simulink subsystem "Autopilot_Commands"  (R2023b)
settings: Solver=VariableStepAuto  StartTime=0.0  StopTime=10.0  RelTol=1e-3
undefined symbols (not defined in the file): Kd, KD_Lateral, Ki, KI_BCL, Kp, KP_BCL, KP_Lateral, KP_TECL, servoLimits
libraries: slpidlib x5, checkpacklib x3, simulink_extras x3, sharedtransform x2
settings Model: Creator=cyber  LastModifiedBy=cyber

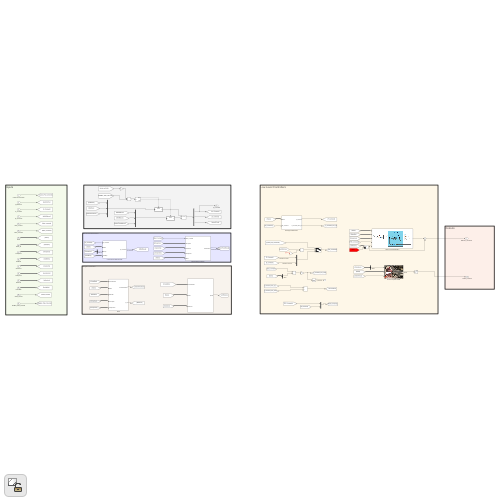
[thumbnail: Simulink's stored preview of the top-level diagram]
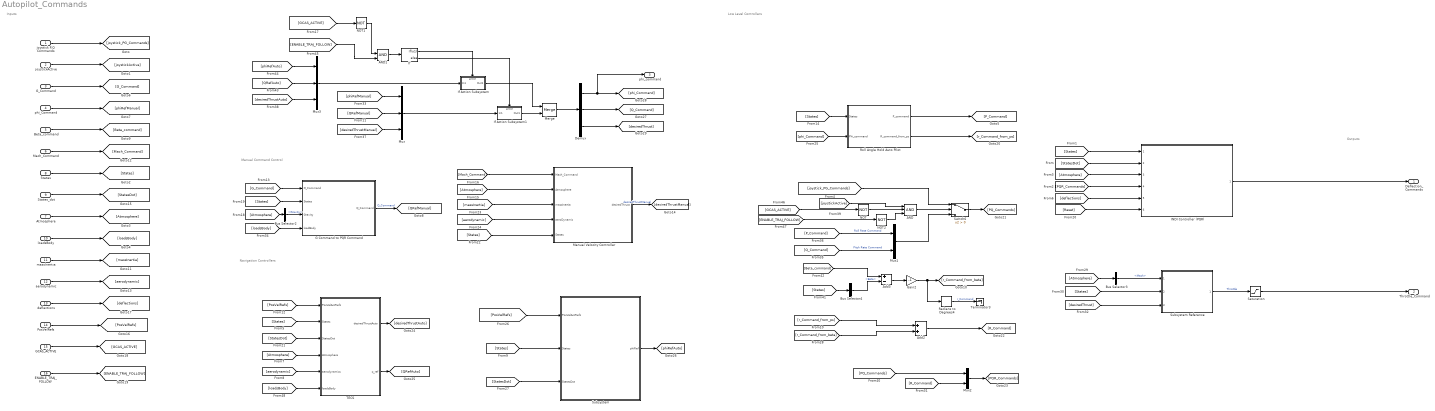
== system Autopilot_Commands ==
  note: Inputs
  note: Manual Command Control
  note: Low Level Controllers
  note: Navigation Controllers
  note: Outputs
  joystick P,Q Commands : Inport
  joystickActive : Inport  Port=2
  G_Command : Inport  Port=3
  phi_Command : Inport  Port=4
  Beta_command : Inport  Port=5
  Mach_Command : Inport  Port=6
  Atmosphere : Inport  Port=7
  States : Inport  Port=8
  States_dot : Inport  Port=9
  loadsBody : Inport  Port=10
  massInertıa : Inport  Port=11
  aerodynamic : Inport  Port=12
  deflections : Inport  Port=13
  PosVelRefs : Inport  Port=14
  GCAS_ACTIVE : Inport  Port=15
  ENABLE_TRAJ_FOLLOW : Inport  Port=16
  AND : Logic  Inputs=3  IconShape=distinctive  AllPortsSameDT=off  OutDataTypeStr=boolean
  AND1 : Logic  IconShape=distinctive  AllPortsSameDT=off  OutDataTypeStr=boolean
  Add2 : Sum
  Add3 : Sum  Inputs=+-
  Bus Selector2 : BusSelector  OutputSignals=Gravity
  Bus Selector3 : BusSelector  OutputSignals=Mach
  Bus Selector4 : BusSelector  OutputSignals=Beta
  Demux : Demux  Outputs=3
  G Command to PQR Command : Subsystem
  Gain2 : Gain  Gain=-1
  INDI Controller (PQR) : Subsystem  ReferencedSubsystem=INDI_Controller_PQR
  If : If  IfExpression=u1
  If Action Subsystem : Subsystem  TreatAsAtomicUnit=on
  If Action Subsystem1 : Subsystem  TreatAsAtomicUnit=on
  Manual Velocity Controller : Subsystem
  Merge : Merge
  Mux : Mux  Inputs=3
  Mux1 : Mux  Inputs=2
  Mux2 : Mux  Inputs=2
  Mux3 : Mux  Inputs=3
  NOT : Logic  Operator=NOT  IconShape=distinctive  AllPortsSameDT=off  OutDataTypeStr=boolean
  NOT1 : Logic  Operator=NOT  IconShape=distinctive  AllPortsSameDT=off  OutDataTypeStr=boolean
  NOT2 : Logic  Operator=NOT  IconShape=distinctive  AllPortsSameDT=off  OutDataTypeStr=boolean
  Radians to Degrees4 : simulink_extras/Transformations/Radians to Degrees
  "Roll Angle Hold Auto Pilot " : Subsystem
  Saturation : Saturate  UpperLimit=100  LowerLimit=-100
  Subsystem : Subsystem
  Subsystem Reference : Subsystem  ReferencedSubsystem=Reverse_Propulsion_Model
  Switch6 : Switch  Criteria=u2 > Threshold  SaturateOnIntegerOverflow=off  InputSameDT=off
  TECS : Subsystem
  Terminator3 : Terminator
  Deflection_Commands : Outport
  Throttle_Command : Outport  Port=2
  phi_command : Outport  Port=3
  wires:
  [PosVelRefs] -> TECS/1(PosVelAccRefs)
  Demux/3 -> [desiredThrust]
  [States] -> G Command to PQR Command/2(States)
  [aerodynamic] -> TECS/5(aerodynamics)
  Saturation/1 -> Throttle_Command/1
  Subsystem/1(phiRef) -> [phiRefAuto]
  If/1 -> If Action Subsystem/Action
  Add3/1 -> Gain2/1
  [phiRefAuto] -> Mux3/1
  [joystick_PG_Commands] -> Switch6/1
  Demux/1 -> [phi_Command], phi_command/1
  deflections/1 -> [deflections]
  [desiredThrustAuto] -> Mux3/3
  Merge/1 -> Demux/1
  If Action Subsystem1/1(Out1) -> Merge/2
  [States] -> "Roll Angle Hold Auto Pilot "/1(States)
  massInertıa/1 -> [massInertia]
  If/2 -> If Action Subsystem1/Action
  If Action Subsystem/1(Out1) -> Merge/1
  loadsBody/1 -> [loadsBody]
  [Mach_Command] -> Manual Velocity Controller/1(Mach_Command)
  [massInertia] -> Manual Velocity Controller/3(massInertia)
  AND1/1 -> If/1
  [States] -> Manual Velocity Controller/5(States)
  Demux/2 -> [Q_Command]
  Mux/1 -> If Action Subsystem1/1(In1)
  [Atmosphere] -> Bus Selector2/1
  Subsystem Reference/1 -> Saturation/1  "Throttle"
  Bus Selector2/1 -> G Command to PQR Command/3(Gravity)  "<Gravity>"
  [Q_Command] -> Mux1/2  "Pitch Rate Command"
  Bus Selector3/1 -> Subsystem Reference/1  "<Mach>"
  [States] -> Subsystem Reference/2
  [phiRefManual] -> Mux/1
  [R_Command] -> Mux2/2
  TECS/2(q_ref) -> [QRefAuto]
  G_Command/1 -> [G_Command]
  [Atmosphere] -> Bus Selector3/1
  [Atmosphere] -> Manual Velocity Controller/2(Atmosphere)
  aerodynamic/1 -> [aerodynamic]
  [PosVelRefs] -> Subsystem/1(PosVelAccRefs)
  G Command to PQR Command/1(Q_Command) -> [QRefManual]  "Q_Command"
  [States] -> Subsystem/2(States)
  [StatesDot] -> TECS/3(StatesDot)
  [Atmosphere] -> TECS/4(Atmosphere)
  Mach_Command/1 -> [Mach_Command]
  [QRefAuto] -> Mux3/2
  [StatesDot] -> Subsystem/3(StatesDot)
  Beta_command/1 -> [Beta_command]
  States_dot/1 -> [StatesDot]
  Switch6/1 -> [PQ_Commands]
  [desiredThrustManual] -> Mux/3
  Mux1/1 -> Switch6/3
  TECS/1(desiredThrustAuto) -> [desiredThrustAuto]
  [G_Command] -> G Command to PQR Command/1(G_Command)
  Atmosphere/1 -> [Atmosphere]
  Gain2/1 -> [r_Command_from_beta], Radians to Degrees4/1
  AND/1 -> Switch6/2
  [P_Command] -> Mux1/1  "Roll Rate Command"
  [loadsBody] -> G Command to PQR Command/4(loadBody)
  States/1 -> [States]
  [desiredThrust] -> Subsystem Reference/3
  joystick P,Q Commands/1 -> [joystick_PG_Commands]
  joystickActive/1 -> [joystickActive]
  phi_Command/1 -> [phiRefManual]
  PosVelRefs/1 -> [PosVelRefs]
  [States] -> TECS/2(States)
  Manual Velocity Controller/1(desiredThrust) -> [desiredThrustManual]  "desiredThrustManual"
  Bus Selector4/1 -> Add3/2  "<Beta>"
  [phi_Command] -> "Roll Angle Hold Auto Pilot "/2(Phi_command)
  "Roll Angle Hold Auto Pilot "/2(R_command_from_ps) -> [r_Command_from_ps]
  [r_Command_from_beta] -> Add2/2
  [QRefManual] -> Mux/2
  [PQ_Commands] -> Mux2/1
  Mux3/1 -> If Action Subsystem/1(In1)
  Add2/1 -> [R_Command]
  "Roll Angle Hold Auto Pilot "/1(P_command) -> [P_Command]
  Radians to Degrees4/1 -> Terminator3/1  "r_Command"
  [States] -> Bus Selector4/1
  [aerodynamic] -> Manual Velocity Controller/4(aeroDynamic)
  [r_Command_from_ps] -> Add2/1
  [Beta_command] -> Add3/1
  Mux2/1 -> [PQR_Commands]
  [GCAS_ACTIVE] -> NOT/1
  NOT/1 -> AND/2
  [joystickActive] -> AND/1
  GCAS_ACTIVE/1 -> [GCAS_ACTIVE]
  [GCAS_ACTIVE] -> NOT1/1
  ENABLE_TRAJ_FOLLOW/1 -> [ENABLE_TRAJ_FOLLOW]
  NOT1/1 -> AND1/1
  [ENABLE_TRAJ_FOLLOW] -> AND1/2
  [ENABLE_TRAJ_FOLLOW] -> NOT2/1
  NOT2/1 -> AND/3
  [loadsBody] -> TECS/6(loadsBody)
  [States] -> INDI Controller (PQR)/1
  [StatesDot] -> INDI Controller (PQR)/2
  [Atmosphere] -> INDI Controller (PQR)/3
  [PQR_Commands] -> INDI Controller (PQR)/4
  [deflections] -> INDI Controller (PQR)/5
  [Reset] -> INDI Controller (PQR)/6
  INDI Controller (PQR)/1 -> Deflection_Commands/1

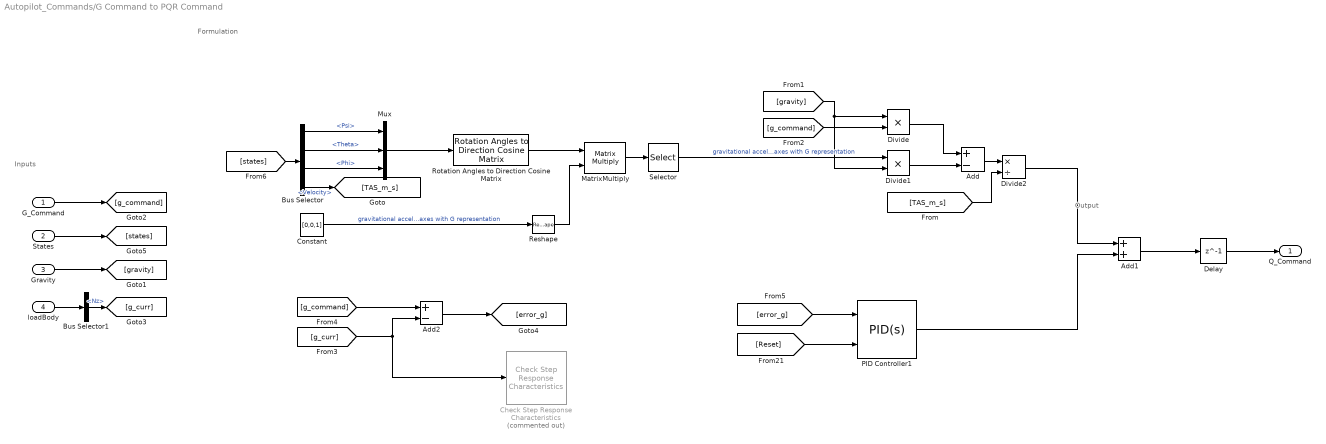
== system Autopilot_Commands/G Command to PQR Command ==
  note: Formulation
  note: Output
  note: Inputs
  G_Command : Inport
  States : Inport  Port=2
  Gravity : Inport  Port=3
  loadBody : Inport  Port=4
  Add : Sum  Inputs=+-
  Add1 : Sum
  Add2 : Sum  Inputs=+-
  Bus Selector : BusSelector  OutputSignals=Psi,Theta,Phi,Velocity
  Bus Selector1 : BusSelector  OutputSignals=Nz
  Check Step Response Characteristics : checkpacklib/Check Step Response  Characteristics  Commented=on  InstantiateOnLoad=on  enabled=off  stopWhenAssertionFail=off  export=off  ViewDlgPos=[]  OpenViewOnLoad=off  LaunchViewOnOpen=off  TimeUnits=seconds  EnableStepResponseBound=on  InitialValue=1  FinalValue=5  StepTime=0  RiseTime=0.5  PercentRise=90  SettlingTime=1.2  PercentSettling=1  PercentOvershoot=5  PercentUndershoot=1
      settings: LibrarySourceBlock=|
      | sdolib/Model Verification/Check Step Response
      | Characteristics
  Constant : Constant  Value=[0,0,1]
  Delay : Delay  DelayLength=1
  Divide : Product  Inputs=**
  Divide1 : Product  Inputs=**
  Divide2 : Product  Inputs=*/
  MatrixMultiply : Product  Multiplication=Matrix(*)
  Mux : Mux  Inputs=3
  PID Controller1 : slpidlib/PID Controller  Controller=PID  Form=Parallel  TimeDomain=Continuous-time  UseExternalTs=off  SampleTime=-1  IntegratorMethod=Forward Euler  FilterMethod=Forward Euler  ControllerParametersSource=internal  P=Kp  I=Ki  UseKiTs=off  D=Kd  N=100  UseFilter=on  TunerSelectOption=Transfer Function Based (PID Tuner App)  InitialConditionSource=internal  InitialConditionForIntegrator=0  InitialConditionForFilter=0  DifferentiatorICPrevScaledInput=0  ExternalReset=either  TrackingMode=off  Kt=1  LimitOutput=off  SatLimitsSource=external  UpperSaturationLimit=inf  LowerSaturationLimit=-inf  LinearizeAsGain=on  AntiWindupMode=clamping  Kb=1  LimitIntegrator=off  UpperIntegratorSaturationLimit=inf  LowerIntegratorSaturationLimit=-inf  POutMin=[]  POutMax=[]  IOutMin=[]  IOutMax=[]  DOutMin=[]  DOutMax=[]  NOutMin=[]  NOutMax=[]  SumOutMin=[]  SumOutMax=[]  SaturationOutMin=[]  SaturationOutMax=[]  PParamMin=[]  PParamMax=[]  IParamMin=[]  IParamMax=[]  DParamMin=[]  DParamMax=[]  NParamMin=[]  NParamMax=[]  KbParamMin=[]  KbParamMax=[]  KtParamMin=[]  KtParamMax=[]  KbOutMin=[]  KbOutMax=[]  KtOutMin=[]  KtOutMax=[]  IntegratorOutMin=[]  IntegratorOutMax=[]  FilterOutMin=[]  FilterOutMax=[]  SumI1OutMin=[]  SumI1OutMax=[]  SumI2OutMin=[]  SumI2OutMax=[]  SumI3OutMin=[]  SumI3OutMax=[]  SumI4OutMin=[]  SumI4OutMax=[]  SumDOutMin=[]  SumDOutMax=[]  DifferentiatorOutMin=[]  DifferentiatorOutMax=[]  FilterDiffOutCoefMin=[]  FilterDiffOutCoefMax=[]  ReciprocalOutMin=[]  ReciprocalOutMax=[]  SumDenOutMin=[]  SumDenOutMax=[]  SumNumOutMin=[]  SumNumOutMax=[]  DivideOutMin=[]  DivideOutMax=[]  UdiffTsProdOutMin=[]  UdiffTsProdOutMax=[]  NTsProdOutMin=[]  NTsProdOutMax=[]  UintegralTsProdOutMin=[]  UintegralTsProdOutMax=[]  UngainTsProdOutMin=[]  UngainTsProdOutMax=[]  ClampingZeroOutDataTypeStr=Inherit: Inherit via back propagation  ClampingZeroOutMin=[]  ClampingZeroOutMax=[]  FilterDenConstantOutDataTypeStr=Inherit: Inherit via back propagation  FilterDenConstantOutMin=[]  FilterDenConstantOutMax=[]  PCopyOutDataTypeStr=Inherit: Inherit via back propagation  PCopyOutMin=[]  PCopyOutMax=[]  NCopyOutDataTypeStr=Inherit: Inherit via back propagation  NCopyOutMin=[]  NCopyOutMax=[]  IntegratorContinuousStateAttributes=''  IntegratorStateMustResolveToSignalObject=off  IntegratorRTWStateStorageClass=Auto  FilterContinuousStateAttributes=''  FilterStateMustResolveToSignalObject=off  FilterRTWStateStorageClass=Auto  ParallelPVariant=InternalParameters  IdealPVariant=Disabled  IVariant=InternalParameters  DVariant=InternalParameters  IntegratorVariant=Continuous  SatVariant=Disabled  AWVariant=Passthrough  PCopyVariant=Disabled  TRVariant=Disabled  FdbkBlocksVariant=Forward  IdealPFdbkVariant=Disabled  SatFdbkVariant=Disabled  DerivativeFilterVariant=ContFilter  NVariant=InternalParameters  NCopyVariant=Disabled  FilterICVariant=InternalICsFilter  IntegratorICVariant=InternalICs  ExternalResetVariant=ExternalReset  TRSumVariant=Passthrough  SumFdbkVariant=Disabled  SumVariant=Sum_PID  TsampFilterVariant=InternalTs  TsampNgainVariant=Passthrough  TsampIntegralVariant=Disabled_SignalSpec  ExternalSaturationOutDataTypeStr=Inherit: Same as second input
  Reshape : Reshape  OutputDimensionality=Column vector (2-D)
  Rotation Angles to Direction Cosine Matrix : sharedtransform/Rotation Angles to Direction Cosine Matrix  rotationOrder=ZYX  aMode=aMode
  Selector : Selector  InputPortWidth=3  IndexOptions=Index vector (dialog)  Indices=3  OutputSizes=1
  Q_Command : Outport
  wires:
  [states] -> Bus Selector/1
  Delay/1 -> Q_Command/1
  Add2/1 -> [error_g]
  [g_curr] -> Add2/2, Check Step Response Characteristics/1
  [g_command] -> Add2/1
  Bus Selector1/1 -> [g_curr]  "<Nz>"
  loadBody/1 -> Bus Selector1/1
  Add1/1 -> Delay/1
  PID Controller1/1 -> Add1/2
  [Reset] -> PID Controller1/2
  [error_g] -> PID Controller1/1
  G_Command/1 -> [g_command]
  Gravity/1 -> [gravity]
  Divide2/1 -> Add1/1
  Divide1/1 -> Add/2
  Divide/1 -> Add/1
  Selector/1 -> Divide1/1  "gravitational acceleration on Body Z axes with G representation"
  Add/1 -> Divide2/1
  [gravity] -> Divide1/2, Divide/1
  Reshape/1 -> MatrixMultiply/2
  [TAS_m_s] -> Divide2/2
  Bus Selector/4 -> [TAS_m_s]  "<Velocity>"
  [g_command] -> Divide/2
  MatrixMultiply/1 -> Selector/1
  Constant/1 -> Reshape/1  "gravitational acceleration on NED axes with G representation"
  Bus Selector/3 -> Mux/3  "<Phi>"
  Bus Selector/1 -> Mux/1  "<Psi>"
  Bus Selector/2 -> Mux/2  "<Theta>"
  Rotation Angles to Direction Cosine Matrix/1 -> MatrixMultiply/1
  Mux/1 -> Rotation Angles to Direction Cosine Matrix/1
  States/1 -> [states]

== system Autopilot_Commands/If Action Subsystem ==
  In1 : Inport
  Action Port : ActionPort
  Out1 : Outport
  wires:
  In1/1 -> Out1/1

== system Autopilot_Commands/If Action Subsystem1 ==
  In1 : Inport
  Action Port : ActionPort
  Out1 : Outport
  wires:
  In1/1 -> Out1/1

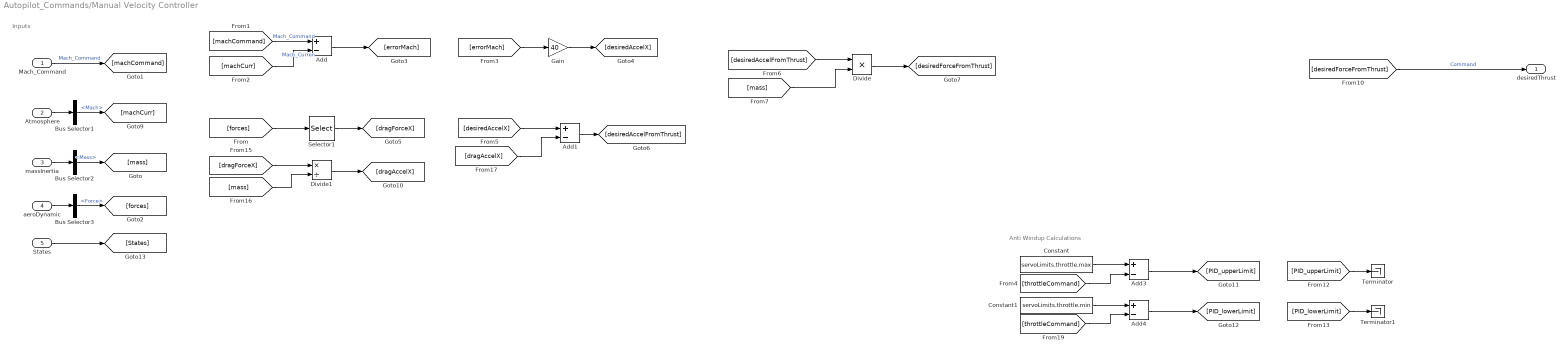
== system Autopilot_Commands/Manual Velocity Controller ==
  note: Inputs
  note: Anti Windup Calculations
  Mach_Command : Inport
  Atmosphere : Inport  Port=2
  massInertia : Inport  Port=3
  aeroDynamic : Inport  Port=4
  States : Inport  Port=5
  Add{,1,3..4} (4 alike) : Sum  Inputs=+-
  Bus Selector1 : BusSelector  OutputSignals=Mach
  Bus Selector2 : BusSelector  OutputSignals=Mass
  Bus Selector3 : BusSelector  OutputSignals=Force
  Constant : Constant  Value=servoLimits.throttle.max
  Constant1 : Constant  Value=servoLimits.throttle.min
  Divide : Product  Inputs=**
  Divide1 : Product  Inputs=*/
  Gain : Gain  Gain=40
  Selector1 : Selector  InputPortWidth=3  IndexOptions=Index vector (dialog)  Indices=1  OutputSizes=1
  Terminator : Terminator
  Terminator1 : Terminator
  desiredThrust : Outport
  wires:
  [PID_lowerLimit] -> Terminator1/1
  [PID_upperLimit] -> Terminator/1
  Atmosphere/1 -> Bus Selector1/1
  Bus Selector1/1 -> [machCurr]  "<Mach>"
  Mach_Command/1 -> [machCommand]  "Mach_Command"
  massInertia/1 -> Bus Selector2/1
  Bus Selector2/1 -> [mass]  "<Mass>"
  aeroDynamic/1 -> Bus Selector3/1
  Bus Selector3/1 -> [forces]  "<Force>"
  [forces] -> Selector1/1
  [machCurr] -> Add/2  "Mach_Curren"
  [machCommand] -> Add/1  "Mach_Command"
  Add/1 -> [errorMach]
  [errorMach] -> Gain/1
  Gain/1 -> [desiredAccelX]
  Selector1/1 -> [dragForceX]
  [desiredAccelX] -> Add1/1
  [dragAccelX] -> Add1/2
  Add1/1 -> [desiredAccelFromThrust]
  [desiredAccelFromThrust] -> Divide/1
  [mass] -> Divide/2
  Divide/1 -> [desiredForceFromThrust]
  States/1 -> [States]
  [dragForceX] -> Divide1/1
  [mass] -> Divide1/2
  Divide1/1 -> [dragAccelX]
  Constant1/1 -> Add4/1
  [throttleCommand] -> Add4/2
  [throttleCommand] -> Add3/2
  Constant/1 -> Add3/1
  Add4/1 -> [PID_lowerLimit]
  Add3/1 -> [PID_upperLimit]
  [desiredForceFromThrust] -> desiredThrust/1  "Command"

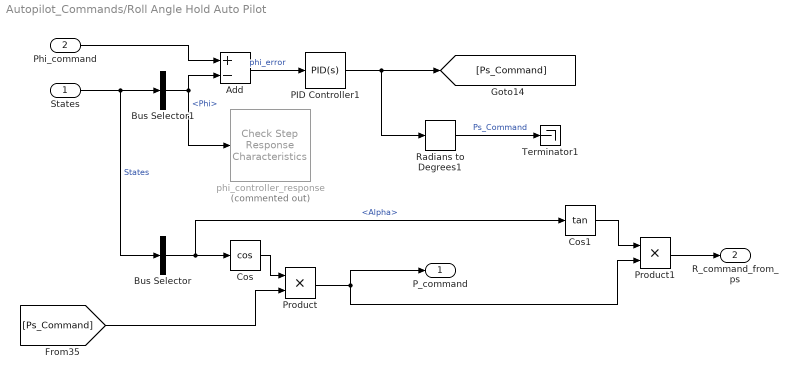
== system Autopilot_Commands/Roll Angle Hold Auto Pilot  ==
  States : Inport
  Phi_command : Inport  Port=2
  Add : Sum  Inputs=+-
  Bus Selector : BusSelector  OutputSignals=Alpha
  Bus Selector1 : BusSelector  OutputSignals=Phi
  Cos : Trigonometry  Operator=cos
  Cos1 : Trigonometry  Operator=tan
  PID Controller1 : slpidlib/PID Controller  Controller=PID  Form=Parallel  TimeDomain=Continuous-time  UseExternalTs=off  SampleTime=-1  IntegratorMethod=Forward Euler  FilterMethod=Forward Euler  ControllerParametersSource=internal  P=1.5  I=0  UseKiTs=off  D=5  N=0  UseFilter=on  TunerSelectOption=Transfer Function Based (PID Tuner App)  InitialConditionSource=internal  InitialConditionForIntegrator=0  InitialConditionForFilter=0  DifferentiatorICPrevScaledInput=0  ExternalReset=none  TrackingMode=off  Kt=1  LimitOutput=off  SatLimitsSource=internal  UpperSaturationLimit=inf  LowerSaturationLimit=-inf  LinearizeAsGain=on  AntiWindupMode=none  Kb=1  LimitIntegrator=off  UpperIntegratorSaturationLimit=inf  LowerIntegratorSaturationLimit=-inf  POutMin=[]  POutMax=[]  IOutMin=[]  IOutMax=[]  DOutMin=[]  DOutMax=[]  NOutMin=[]  NOutMax=[]  SumOutMin=[]  SumOutMax=[]  SaturationOutMin=[]  SaturationOutMax=[]  PParamMin=[]  PParamMax=[]  IParamMin=[]  IParamMax=[]  DParamMin=[]  DParamMax=[]  NParamMin=[]  NParamMax=[]  KbParamMin=[]  KbParamMax=[]  KtParamMin=[]  KtParamMax=[]  KbOutMin=[]  KbOutMax=[]  KtOutMin=[]  KtOutMax=[]  IntegratorOutMin=[]  IntegratorOutMax=[]  FilterOutMin=[]  FilterOutMax=[]  SumI1OutMin=[]  SumI1OutMax=[]  SumI2OutMin=[]  SumI2OutMax=[]  SumI3OutMin=[]  SumI3OutMax=[]  SumI4OutMin=[]  SumI4OutMax=[]  SumDOutMin=[]  SumDOutMax=[]  DifferentiatorOutMin=[]  DifferentiatorOutMax=[]  FilterDiffOutCoefMin=[]  FilterDiffOutCoefMax=[]  ReciprocalOutMin=[]  ReciprocalOutMax=[]  SumDenOutMin=[]  SumDenOutMax=[]  SumNumOutMin=[]  SumNumOutMax=[]  DivideOutMin=[]  DivideOutMax=[]  UdiffTsProdOutMin=[]  UdiffTsProdOutMax=[]  NTsProdOutMin=[]  NTsProdOutMax=[]  UintegralTsProdOutMin=[]  UintegralTsProdOutMax=[]  UngainTsProdOutMin=[]  UngainTsProdOutMax=[]  ClampingZeroOutDataTypeStr=Inherit: Inherit via back propagation  ClampingZeroOutMin=[]  ClampingZeroOutMax=[]  FilterDenConstantOutDataTypeStr=Inherit: Inherit via back propagation  FilterDenConstantOutMin=[]  FilterDenConstantOutMax=[]  PCopyOutDataTypeStr=Inherit: Inherit via back propagation  PCopyOutMin=[]  PCopyOutMax=[]  NCopyOutDataTypeStr=Inherit: Inherit via back propagation  NCopyOutMin=[]  NCopyOutMax=[]  IntegratorContinuousStateAttributes=''  IntegratorStateMustResolveToSignalObject=off  IntegratorRTWStateStorageClass=Auto  FilterContinuousStateAttributes=''  FilterStateMustResolveToSignalObject=off  FilterRTWStateStorageClass=Auto  ParallelPVariant=InternalParameters  IdealPVariant=Disabled  IVariant=InternalParameters  DVariant=InternalParameters  IntegratorVariant=Continuous  SatVariant=Disabled  AWVariant=Passthrough  PCopyVariant=Disabled  TRVariant=Disabled  FdbkBlocksVariant=Forward  IdealPFdbkVariant=Disabled  SatFdbkVariant=Disabled  DerivativeFilterVariant=ContFilter  NVariant=InternalParameters  NCopyVariant=Disabled  FilterICVariant=InternalICsFilter  IntegratorICVariant=InternalICs  ExternalResetVariant=Disabled  TRSumVariant=Passthrough  SumFdbkVariant=Disabled  SumVariant=Sum_PID  TsampFilterVariant=InternalTs  TsampNgainVariant=Passthrough  TsampIntegralVariant=Disabled_SignalSpec  ExternalSaturationOutDataTypeStr=Inherit: Same as second input
  Product : Product
  Product1 : Product
  Radians to Degrees1 : simulink_extras/Transformations/Radians to Degrees
  Terminator1 : Terminator
  phi_controller_response : checkpacklib/Check Step Response  Characteristics  Commented=on  InstantiateOnLoad=on  enabled=off  stopWhenAssertionFail=off  export=off  ViewDlgPos=[]  OpenViewOnLoad=off  LaunchViewOnOpen=off  TimeUnits=seconds  EnableStepResponseBound=on  InitialValue=0  FinalValue=pi/2  StepTime=0  RiseTime=2  PercentRise=90  SettlingTime=3  PercentSettling=2  PercentOvershoot=3  PercentUndershoot=1
      settings: LibrarySourceBlock=|
      | sdolib/Model Verification/Check Step Response
      | Characteristics
  P_command : Outport
  R_command_from_ps : Outport  Port=2
  wires:
  Product1/1 -> R_command_from_ps/1
  Add/1 -> PID Controller1/1  "phi_error"
  Bus Selector1/1 -> Add/2, phi_controller_response/1  "<Phi>"
  Cos/1 -> Product/1
  Bus Selector/1 -> Cos/1, Cos1/1  "<Alpha>"
  Phi_command/1 -> Add/1
  Radians to Degrees1/1 -> Terminator1/1  "Ps_Command"
  Cos1/1 -> Product1/1
  Product/1 -> Product1/2, P_command/1
  PID Controller1/1 -> Radians to Degrees1/1, [Ps_Command]
  States/1 -> Bus Selector1/1, Bus Selector/1  "States"
  [Ps_Command] -> Product/2

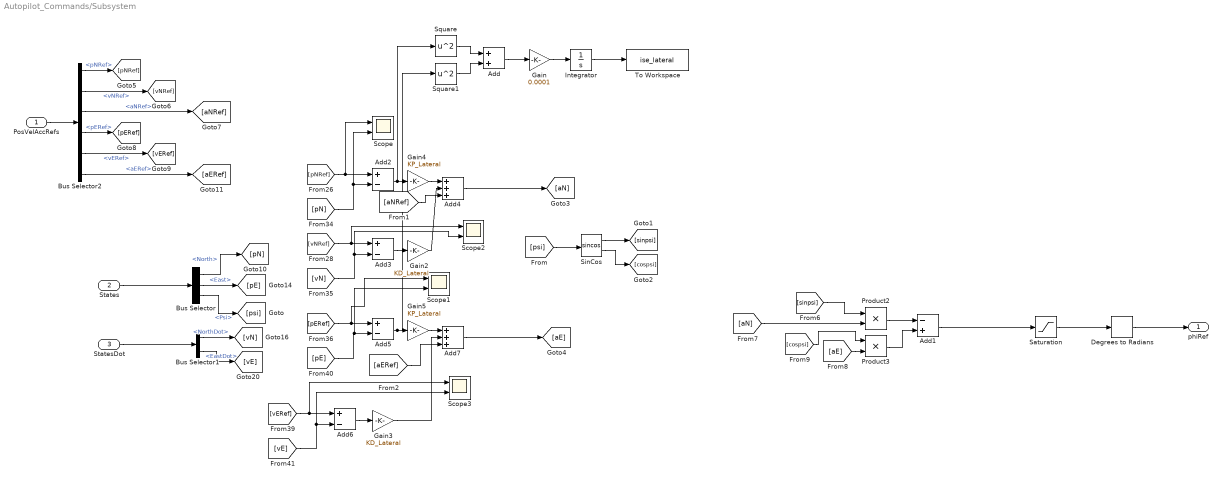
== system Autopilot_Commands/Subsystem ==
  PosVelAccRefs : Inport
  States : Inport  Port=2
  StatesDot : Inport  Port=3
  Add : Sum
  Add1 : Sum  Inputs=-+
  Add{2..3,5..6} (4 alike) : Sum  Inputs=+-
  Add4 : Sum  Inputs=+++
  Add7 : Sum  Inputs=+++
  Bus Selector : BusSelector  OutputSignals=North,East,Psi
  Bus Selector1 : BusSelector  OutputSignals=NorthDot,EastDot
  Bus Selector2 : BusSelector  OutputSignals=pNRef,vNRef,aNRef,pERef,vERef,aERef
  Degrees to Radians : simulink_extras/Transformations/Degrees to Radians
  Gain : Gain  Gain=0.0001
  Gain2 : Gain  Gain=KD_Lateral
  Gain3 : Gain  Gain=KD_Lateral
  Gain4 : Gain  Gain=KP_Lateral
  Gain5 : Gain  Gain=KP_Lateral
  Integrator : Integrator
  Product2 : Product
  Product3 : Product
  Saturation : Saturate  UpperLimit=60  LowerLimit=-60
  Scope{,1..3} (4 alike) : Scope  NumInputPorts=2
  SinCos : Trigonometry  Operator=sincos
  Square : Math  Operator=square
  Square1 : Math  Operator=square
  To Workspace : ToWorkspace  VariableName=ise_lateral  SaveFormat=Timeseries  SampleTime=-1
  phiRef : Outport
  wires:
  [aERef] -> Add7/3
  [aNRef] -> Add4/3
  Bus Selector2/6 -> [aERef]  "<aERef>"
  Bus Selector2/5 -> [vERef]  "<vERef>"
  Bus Selector2/4 -> [pERef]  "<pERef>"
  Bus Selector2/3 -> [aNRef]  "<aNRef>"
  Bus Selector2/2 -> [vNRef]  "<vNRef>"
  Bus Selector2/1 -> [pNRef]  "<pNRef>"
  PosVelAccRefs/1 -> Bus Selector2/1
  Add1/1 -> Saturation/1
  Gain/1 -> Integrator/1
  Integrator/1 -> To Workspace/1
  Square1/1 -> Add/2
  Square/1 -> Add/1
  Add/1 -> Gain/1
  Gain5/1 -> Add7/1
  Gain4/1 -> Add4/1
  Degrees to Radians/1 -> phiRef/1
  [pERef] -> Add5/1, Scope1/1
  [pE] -> Add5/2, Scope1/2
  Gain3/1 -> Add7/2
  Gain2/1 -> Add4/2
  Add4/1 -> [aN]
  Saturation/1 -> Degrees to Radians/1
  [aN] -> Product2/2
  [sinpsi] -> Product2/1
  [aE] -> Product3/2
  Product2/1 -> Add1/1
  [cospsi] -> Product3/1
  Product3/1 -> Add1/2
  SinCos/2 -> [cospsi]
  SinCos/1 -> [sinpsi]
  [psi] -> SinCos/1
  Bus Selector/3 -> [psi]  "<Psi>"
  StatesDot/1 -> Bus Selector1/1
  States/1 -> Bus Selector/1
  Bus Selector/1 -> [pN]  "<North>"
  Add5/1 -> Gain5/1, Square1/1
  [vERef] -> Add6/1, Scope3/1
  [vE] -> Add6/2, Scope3/2
  Bus Selector1/1 -> [vN]  "<NorthDot>"
  [pNRef] -> Add2/1, Scope/1
  [vNRef] -> Add3/1, Scope2/1
  [pN] -> Add2/2, Scope/2
  Bus Selector/2 -> [pE]  "<East>"
  [vN] -> Add3/2, Scope2/2
  Add6/1 -> Gain3/1
  Add3/1 -> Gain2/1
  Add7/1 -> [aE]
  Bus Selector1/2 -> [vE]  "<EastDot>"
  Add2/1 -> Gain4/1, Square/1

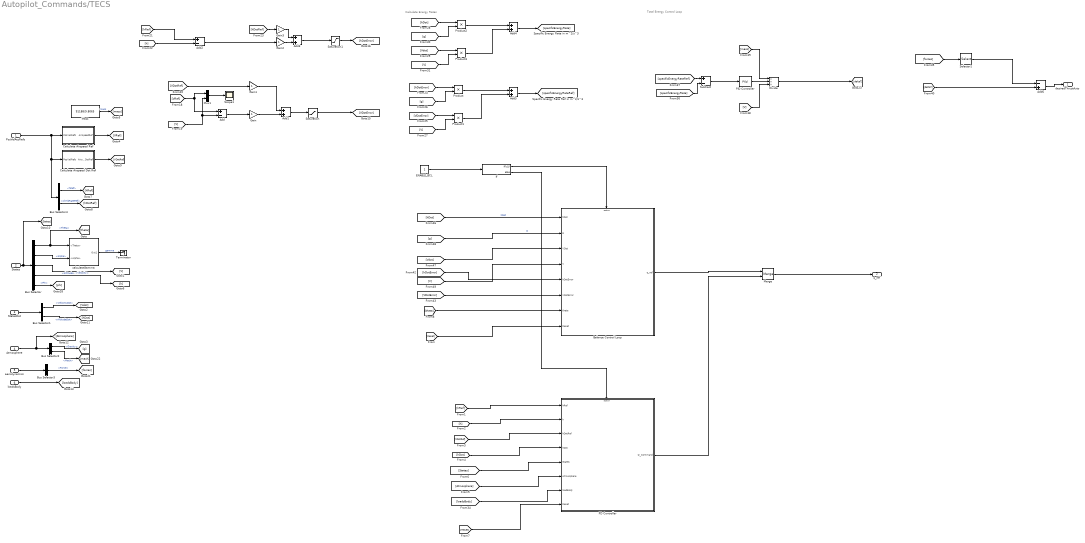
== system Autopilot_Commands/TECS ==
  note: Calculate Energy Rates
  note: Total Energy Control Loop
  PosVelAccRefs : Inport
  States : Inport  Port=2
  StatesDot : Inport  Port=3
  Atmosphere : Inport  Port=4
  aerodynamics : Inport  Port=5
  loadsBody : Inport  Port=6
  Add : Sum  Inputs=+-
  Add{1,3..5} (4 alike) : Sum
  Add2 : Sum  Inputs=+-
  Add6 : Sum  Inputs=-+
  Balance Control Loop : Subsystem
  Bus Selector : BusSelector  OutputSignals=Theta,Alpha,Velocity,Altitude,Phi
  Bus Selector1 : BusSelector  OutputSignals=VelocityDot,AltitudeDot
  Bus Selector2 : BusSelector  OutputSignals=Gravity,Mach
  Bus Selector3 : BusSelector  OutputSignals=Force
  Bus Selector4 : BusSelector  OutputSignals=hRef,climbRateRef
  Calculate Airspeed Dot Ref : Subsystem
  Calculate Airspeed Ref : Subsystem
  Divide : Product  Inputs=**/
  ENABLE_BCL : Constant
      settings: OpenFcn=|
      | val = get_param(gcb,'Value')
      | 
      | switch val
      | case '1'
      | set_param(gcb,'Value','0')
      | set_param(gcb,'BackGroundColor','red')
      | otherwise
      | set_param(gcb,'Value','1')
      | set_param(gcb,'BackGroundColor','green')
      | end
  Gain{,1..3} (4 alike) : Gain
  If : If  IfExpression=u1
  Mass : Constant  Value=91188/9.8065
  Merge : Merge
  Mux1 : Mux  Inputs=2
  PD Controller : Subsystem
  PID Controller : slpidlib/PID Controller  Controller=PI  Form=Parallel  TimeDomain=Continuous-time  UseExternalTs=off  SampleTime=-1  IntegratorMethod=Forward Euler  FilterMethod=Forward Euler  ControllerParametersSource=internal  P=KP_TECL  I=0  UseKiTs=off  D=0  N=100  UseFilter=on  TunerSelectOption=Transfer Function Based (PID Tuner App)  InitialConditionSource=internal  InitialConditionForIntegrator=0  InitialConditionForFilter=0  DifferentiatorICPrevScaledInput=0  ExternalReset=none  TrackingMode=off  Kt=1  LimitOutput=off  SatLimitsSource=internal  UpperSaturationLimit=inf  LowerSaturationLimit=-inf  LinearizeAsGain=on  AntiWindupMode=none  Kb=1  LimitIntegrator=off  UpperIntegratorSaturationLimit=inf  LowerIntegratorSaturationLimit=-inf  POutMin=[]  POutMax=[]  IOutMin=[]  IOutMax=[]  DOutMin=[]  DOutMax=[]  NOutMin=[]  NOutMax=[]  SumOutMin=[]  SumOutMax=[]  SaturationOutMin=[]  SaturationOutMax=[]  PParamMin=[]  PParamMax=[]  IParamMin=[]  IParamMax=[]  DParamMin=[]  DParamMax=[]  NParamMin=[]  NParamMax=[]  KbParamMin=[]  KbParamMax=[]  KtParamMin=[]  KtParamMax=[]  KbOutMin=[]  KbOutMax=[]  KtOutMin=[]  KtOutMax=[]  IntegratorOutMin=[]  IntegratorOutMax=[]  FilterOutMin=[]  FilterOutMax=[]  SumI1OutMin=[]  SumI1OutMax=[]  SumI2OutMin=[]  SumI2OutMax=[]  SumI3OutMin=[]  SumI3OutMax=[]  SumI4OutMin=[]  SumI4OutMax=[]  SumDOutMin=[]  SumDOutMax=[]  DifferentiatorOutMin=[]  DifferentiatorOutMax=[]  FilterDiffOutCoefMin=[]  FilterDiffOutCoefMax=[]  ReciprocalOutMin=[]  ReciprocalOutMax=[]  SumDenOutMin=[]  SumDenOutMax=[]  SumNumOutMin=[]  SumNumOutMax=[]  DivideOutMin=[]  DivideOutMax=[]  UdiffTsProdOutMin=[]  UdiffTsProdOutMax=[]  NTsProdOutMin=[]  NTsProdOutMax=[]  UintegralTsProdOutMin=[]  UintegralTsProdOutMax=[]  UngainTsProdOutMin=[]  UngainTsProdOutMax=[]  ClampingZeroOutDataTypeStr=Inherit: Inherit via back propagation  ClampingZeroOutMin=[]  ClampingZeroOutMax=[]  FilterDenConstantOutDataTypeStr=Inherit: Inherit via back propagation  FilterDenConstantOutMin=[]  FilterDenConstantOutMax=[]  PCopyOutDataTypeStr=Inherit: Inherit via back propagation  PCopyOutMin=[]  PCopyOutMax=[]  NCopyOutDataTypeStr=Inherit: Inherit via back propagation  NCopyOutMin=[]  NCopyOutMax=[]  IntegratorContinuousStateAttributes=''  IntegratorStateMustResolveToSignalObject=off  IntegratorRTWStateStorageClass=Auto  FilterContinuousStateAttributes=''  FilterStateMustResolveToSignalObject=off  FilterRTWStateStorageClass=Auto  ParallelPVariant=InternalParameters  IdealPVariant=Disabled  IVariant=InternalParameters  DVariant=Disabled  IntegratorVariant=Continuous  SatVariant=Disabled  AWVariant=Passthrough  PCopyVariant=Disabled  TRVariant=Disabled  FdbkBlocksVariant=Forward  IdealPFdbkVariant=Disabled  SatFdbkVariant=Disabled  DerivativeFilterVariant=Disabled  NVariant=Disabled  NCopyVariant=Disabled_SignalSpec  FilterICVariant=Disabled  IntegratorICVariant=InternalICs  ExternalResetVariant=Disabled  TRSumVariant=Passthrough  SumFdbkVariant=Disabled  SumVariant=Sum_PI  TsampFilterVariant=InternalTs  TsampNgainVariant=Passthrough  TsampIntegralVariant=Disabled_SignalSpec  ExternalSaturationOutDataTypeStr=Inherit: Same as second input
  Product{,1..3} (4 alike) : Product
  Saturation : Saturate  UpperLimit=10  LowerLimit=-10
  Saturation1 : Saturate  UpperLimit=20  LowerLimit=-20
  Scope1 : Scope
  Selector1 : Selector  InputPortWidth=3  IndexOptions=Index vector (dialog)  Indices=1  OutputSizes=1
  Subtract : Sum  Inputs=+-
  Terminator : Terminator
  calculateGamma : Subsystem
  desiredThrustAuto : Outport
  q_ref : Outport  Port=2
  wires:
  [theta] -> Balance Control Loop/7(theta)
  [Reset] -> PD Controller/8(Reset)
  [Reset] -> Balance Control Loop/8(Reset)
  loadsBody/1 -> [loadsBody]
  PD Controller/1(Q_Command) -> Merge/2
  [loadsBody] -> PD Controller/7(loadBody)
  [Atmosphere] -> PD Controller/6(Atmosphere)
  [States] -> PD Controller/5(States)
  [hDot] -> PD Controller/4(hDot)
  [hDotRef] -> PD Controller/3(hDotRef)
  [h] -> PD Controller/2(h)
  [hRef] -> PD Controller/1(hRef)
  If/2 -> PD Controller/Action
  Merge/1 -> q_ref/1
  If/1 -> Balance Control Loop/Action
  ENABLE_BCL/1 -> If/1
  Balance Control Loop/1(q_ref) -> Merge/1
  [VDotError] -> Balance Control Loop/6(VDotError)
  [hDotError] -> Balance Control Loop/5(hDotError)
  [V] -> Balance Control Loop/4(V)
  [Vdot] -> Balance Control Loop/3(VDot)
  [g] -> Balance Control Loop/2(g)  "g"
  [hDot] -> Balance Control Loop/1(hDot)  "hDot"
  Calculate Airspeed Dot Ref/1(AirspeedDotRef) -> [VDotRef]
  PosVelAccRefs/1 -> Calculate Airspeed Ref/1(PosVelRefs), Bus Selector4/1, Calculate Airspeed Dot Ref/1(PosVelRefs)
  Bus Selector4/2 -> [hDotRef]  "<climbRateRef>"
  Bus Selector4/1 -> [hRef]  "<hRef>"
  Calculate Airspeed Ref/1(AirspeedRef) -> [VRef]
  [VRef] -> Add/1, Mux1/1
  [V] -> Mux1/2, Add/2
  Mux1/1 -> Scope1/1
  Subtract/1 -> PID Controller/1
  Divide/1 -> [deltaT]
  PID Controller/1 -> Divide/2
  Bus Selector/5 -> [phi]  "<Phi>"
  Add6/1 -> desiredThrustAuto/1
  Selector1/1 -> Add6/1
  [deltaT] -> Add6/2
  [mass] -> Divide/1
  [V] -> Divide/3
  [specificEnergyRate] -> Subtract/2
  [specificEnergyRateRef] -> Subtract/1
  Bus Selector2/2 -> [mach]  "<Mach>"
  [forces] -> Selector1/1
  Bus Selector3/1 -> [forces]  "<Force>"
  aerodynamics/1 -> Bus Selector3/1
  Add5/1 -> [specificEnergyRateRef]
  Add4/1 -> [specificEnergyRate]
  [hDot] -> Product2/1
  [g] -> Product2/2
  Product2/1 -> Add4/1
  [Vdot] -> Product3/1
  [V] -> Product3/2
  Product3/1 -> Add4/2
  Product1/1 -> Add5/2
  [V] -> Product1/2
  [VDotError] -> Product1/1
  Product/1 -> Add5/1
  [g] -> Product/2
  [hDotError] -> Product/1
  Saturation1/1 -> [hDotError]
  Add3/1 -> Saturation1/1
  Gain3/1 -> Add3/1
  [hDotRef] -> Gain3/1
  Gain2/1 -> Add3/2
  Add2/1 -> Gain2/1
  [h] -> Add2/2
  Saturation/1 -> [VDotError]
  [hRef] -> Add2/1
  Add1/1 -> Saturation/1
  Gain1/1 -> Add1/1
  [VDotRef] -> Gain1/1
  Gain/1 -> Add1/2
  Add/1 -> Gain/1
  Bus Selector1/2 -> [hDot]  "<AltitudeDot>"
  Bus Selector/4 -> [h]  "<Altitude>"
  Mass/1 -> [mass]  "mass"
  Bus Selector2/1 -> [g]  "<Gravity>"
  Atmosphere/1 -> Bus Selector2/1, [Atmosphere]
  Bus Selector1/1 -> [Vdot]  "<VelocityDot>"
  StatesDot/1 -> Bus Selector1/1
  Bus Selector/3 -> [V]  "<Velocity>"
  calculateGamma/1(Out1) -> Terminator/1  "gamma"
  States/1 -> Bus Selector/1, [States]
  Bus Selector/1 -> calculateGamma/1(<Theta>), [theta]  "<Theta>"
  Bus Selector/2 -> calculateGamma/2(<Alpha>)  "<Alpha>"

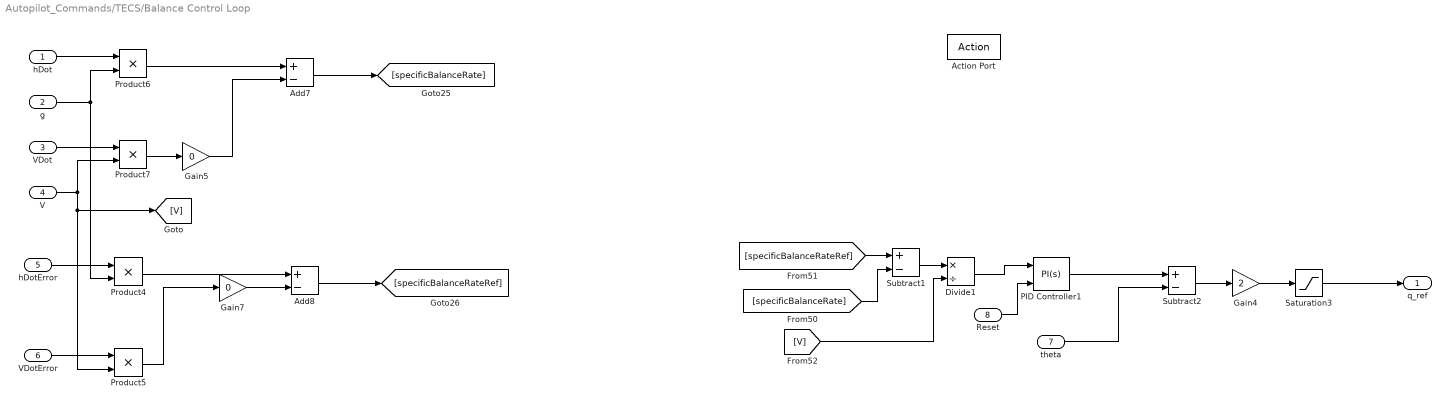
== system Autopilot_Commands/TECS/Balance Control Loop ==
  hDot : Inport
  g : Inport  Port=2
  VDot : Inport  Port=3
  V : Inport  Port=4
  hDotError : Inport  Port=5
  VDotError : Inport  Port=6
  theta : Inport  Port=7
  Reset : Inport  Port=8
  Action Port : ActionPort
  Add7 : Sum  Inputs=+-
  Add8 : Sum  Inputs=+-
  Divide1 : Product  Inputs=*/
  Gain4 : Gain  Gain=2
  Gain5 : Gain  Gain=0
  Gain7 : Gain  Gain=0
  PID Controller1 : slpidlib/PID Controller  Controller=PI  Form=Parallel  TimeDomain=Continuous-time  UseExternalTs=off  SampleTime=-1  IntegratorMethod=Forward Euler  FilterMethod=Forward Euler  ControllerParametersSource=internal  P=KP_BCL  I=KI_BCL  UseKiTs=off  D=0  N=100  UseFilter=on  TunerSelectOption=Transfer Function Based (PID Tuner App)  InitialConditionSource=internal  InitialConditionForIntegrator=0  InitialConditionForFilter=0  DifferentiatorICPrevScaledInput=0  ExternalReset=either  TrackingMode=off  Kt=1  LimitOutput=off  SatLimitsSource=internal  UpperSaturationLimit=inf  LowerSaturationLimit=-inf  LinearizeAsGain=on  AntiWindupMode=none  Kb=1  LimitIntegrator=off  UpperIntegratorSaturationLimit=inf  LowerIntegratorSaturationLimit=-inf  POutMin=[]  POutMax=[]  IOutMin=[]  IOutMax=[]  DOutMin=[]  DOutMax=[]  NOutMin=[]  NOutMax=[]  SumOutMin=[]  SumOutMax=[]  SaturationOutMin=[]  SaturationOutMax=[]  PParamMin=[]  PParamMax=[]  IParamMin=[]  IParamMax=[]  DParamMin=[]  DParamMax=[]  NParamMin=[]  NParamMax=[]  KbParamMin=[]  KbParamMax=[]  KtParamMin=[]  KtParamMax=[]  KbOutMin=[]  KbOutMax=[]  KtOutMin=[]  KtOutMax=[]  IntegratorOutMin=[]  IntegratorOutMax=[]  FilterOutMin=[]  FilterOutMax=[]  SumI1OutMin=[]  SumI1OutMax=[]  SumI2OutMin=[]  SumI2OutMax=[]  SumI3OutMin=[]  SumI3OutMax=[]  SumI4OutMin=[]  SumI4OutMax=[]  SumDOutMin=[]  SumDOutMax=[]  DifferentiatorOutMin=[]  DifferentiatorOutMax=[]  FilterDiffOutCoefMin=[]  FilterDiffOutCoefMax=[]  ReciprocalOutMin=[]  ReciprocalOutMax=[]  SumDenOutMin=[]  SumDenOutMax=[]  SumNumOutMin=[]  SumNumOutMax=[]  DivideOutMin=[]  DivideOutMax=[]  UdiffTsProdOutMin=[]  UdiffTsProdOutMax=[]  NTsProdOutMin=[]  NTsProdOutMax=[]  UintegralTsProdOutMin=[]  UintegralTsProdOutMax=[]  UngainTsProdOutMin=[]  UngainTsProdOutMax=[]  ClampingZeroOutDataTypeStr=Inherit: Inherit via back propagation  ClampingZeroOutMin=[]  ClampingZeroOutMax=[]  FilterDenConstantOutDataTypeStr=Inherit: Inherit via back propagation  FilterDenConstantOutMin=[]  FilterDenConstantOutMax=[]  PCopyOutDataTypeStr=Inherit: Inherit via back propagation  PCopyOutMin=[]  PCopyOutMax=[]  NCopyOutDataTypeStr=Inherit: Inherit via back propagation  NCopyOutMin=[]  NCopyOutMax=[]  IntegratorContinuousStateAttributes=''  IntegratorStateMustResolveToSignalObject=off  IntegratorRTWStateStorageClass=Auto  FilterContinuousStateAttributes=''  FilterStateMustResolveToSignalObject=off  FilterRTWStateStorageClass=Auto  ParallelPVariant=InternalParameters  IdealPVariant=Disabled  IVariant=InternalParameters  DVariant=Disabled  IntegratorVariant=Continuous  SatVariant=Disabled  AWVariant=Passthrough  PCopyVariant=Disabled  TRVariant=Disabled  FdbkBlocksVariant=Forward  IdealPFdbkVariant=Disabled  SatFdbkVariant=Disabled  DerivativeFilterVariant=Disabled  NVariant=Disabled  NCopyVariant=Disabled_SignalSpec  FilterICVariant=Disabled  IntegratorICVariant=InternalICs  ExternalResetVariant=ExternalReset  TRSumVariant=Passthrough  SumFdbkVariant=Disabled  SumVariant=Sum_PI  TsampFilterVariant=InternalTs  TsampNgainVariant=Passthrough  TsampIntegralVariant=Disabled_SignalSpec  ExternalSaturationOutDataTypeStr=Inherit: Same as second input
  Product{4..7} (4 alike) : Product
  Saturation3 : Saturate  UpperLimit=20*pi/180  LowerLimit=-20*pi/180
  Subtract1 : Sum  Inputs=+-
  Subtract2 : Sum  Inputs=+-
  q_ref : Outport
  wires:
  Reset/1 -> PID Controller1/2
  VDot/1 -> Product7/1
  hDotError/1 -> Product4/1
  hDot/1 -> Product6/1
  [specificBalanceRate] -> Subtract1/2
  [V] -> Divide1/2
  Gain7/1 -> Add8/2
  theta/1 -> Subtract2/2
  g/1 -> Product4/2, Product6/2
  V/1 -> Product7/2, Product5/2, [V]
  Subtract2/1 -> Gain4/1
  Subtract1/1 -> Divide1/1
  Product6/1 -> Add7/1
  Product4/1 -> Add8/1
  PID Controller1/1 -> Subtract2/1
  Divide1/1 -> PID Controller1/1
  Product7/1 -> Gain5/1
  Saturation3/1 -> q_ref/1
  VDotError/1 -> Product5/1
  Add7/1 -> [specificBalanceRate]
  [specificBalanceRateRef] -> Subtract1/1
  Gain4/1 -> Saturation3/1
  Add8/1 -> [specificBalanceRateRef]
  Gain5/1 -> Add7/2
  Product5/1 -> Gain7/1

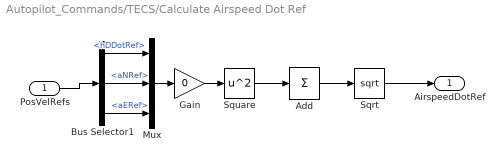
== system Autopilot_Commands/TECS/Calculate Airspeed Dot Ref ==
  PosVelRefs : Inport
  Add : Sum  Inputs=+
  Bus Selector1 : BusSelector  OutputSignals=hDDotRef,aNRef,aERef
  Gain : Gain  Gain=0
  Mux : Mux  Inputs=3
  Sqrt : Sqrt
  Square : Math  Operator=square
  AirspeedDotRef : Outport
  wires:
  Gain/1 -> Square/1
  Bus Selector1/3 -> Mux/3  "<aERef>"
  Bus Selector1/2 -> Mux/2  "<aNRef>"
  Bus Selector1/1 -> Mux/1  "<hDDotRef>"
  Mux/1 -> Gain/1
  Sqrt/1 -> AirspeedDotRef/1
  Square/1 -> Add/1
  Add/1 -> Sqrt/1
  PosVelRefs/1 -> Bus Selector1/1

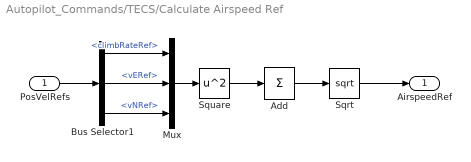
== system Autopilot_Commands/TECS/Calculate Airspeed Ref ==
  PosVelRefs : Inport
  Add : Sum  Inputs=+
  Bus Selector1 : BusSelector  OutputSignals=climbRateRef,vERef,vNRef
  Mux : Mux  Inputs=3
  Sqrt : Sqrt
  Square : Math  Operator=square
  AirspeedRef : Outport
  wires:
  PosVelRefs/1 -> Bus Selector1/1
  Add/1 -> Sqrt/1
  Bus Selector1/1 -> Mux/1  "<climbRateRef>"
  Square/1 -> Add/1
  Sqrt/1 -> AirspeedRef/1
  Bus Selector1/2 -> Mux/2  "<vERef>"
  Mux/1 -> Square/1
  Bus Selector1/3 -> Mux/3  "<vNRef>"

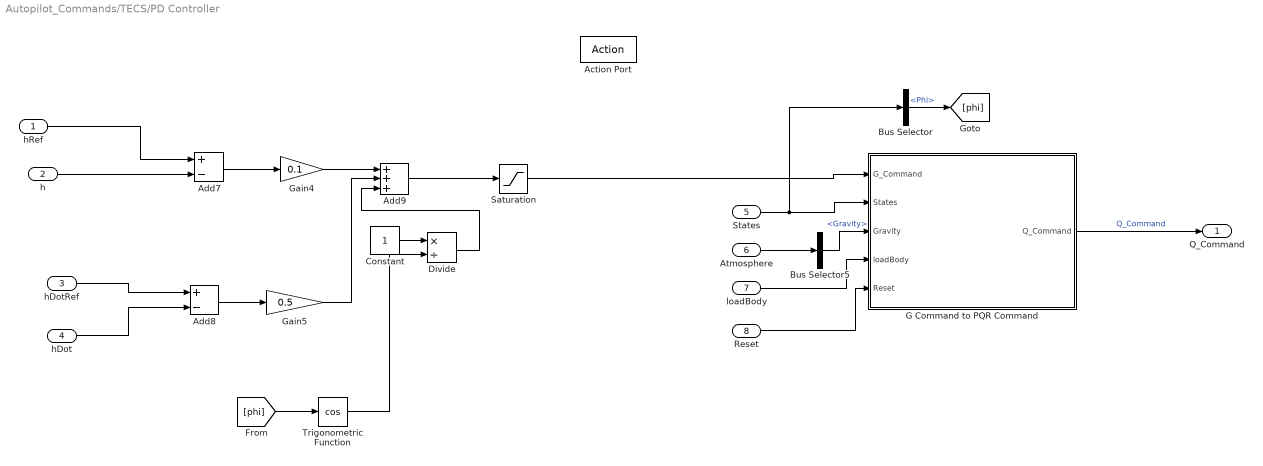
== system Autopilot_Commands/TECS/PD Controller ==
  hRef : Inport
  h : Inport  Port=2
  hDotRef : Inport  Port=3
  hDot : Inport  Port=4
  States : Inport  Port=5
  Atmosphere : Inport  Port=6
  loadBody : Inport  Port=7
  Reset : Inport  Port=8
  Action Port : ActionPort
  Add7 : Sum  Inputs=+-
  Add8 : Sum  Inputs=+-
  Add9 : Sum  Inputs=+++
  Bus Selector : BusSelector  OutputSignals=Phi
  Bus Selector5 : BusSelector  OutputSignals=Gravity
  Constant : Constant
  Divide : Product  Inputs=*/
  G Command to PQR Command : Subsystem
  Gain4 : Gain  Gain=0.1
  Gain5 : Gain  Gain=0.5
  Saturation : Saturate  UpperLimit=5  LowerLimit=-3
  Trigonometric Function : Trigonometry  Operator=cos
  Q_Command : Outport
  wires:
  Divide/1 -> Add9/3
  Constant/1 -> Divide/1
  Trigonometric Function/1 -> Divide/2
  [phi] -> Trigonometric Function/1
  Bus Selector/1 -> [phi]  "<Phi>"
  Saturation/1 -> G Command to PQR Command/1(G_Command)
  Reset/1 -> G Command to PQR Command/5(Reset)
  hRef/1 -> Add7/1
  h/1 -> Add7/2
  hDot/1 -> Add8/2
  Atmosphere/1 -> Bus Selector5/1
  loadBody/1 -> G Command to PQR Command/4(loadBody)
  Add8/1 -> Gain5/1
  Gain5/1 -> Add9/2
  G Command to PQR Command/1(Q_Command) -> Q_Command/1  "Q_Command"
  Bus Selector5/1 -> G Command to PQR Command/3(Gravity)  "<Gravity>"
  Add9/1 -> Saturation/1
  States/1 -> G Command to PQR Command/2(States), Bus Selector/1
  Add7/1 -> Gain4/1
  Gain4/1 -> Add9/1
  hDotRef/1 -> Add8/1

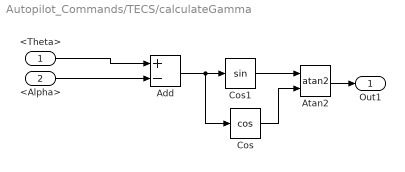
== system Autopilot_Commands/TECS/calculateGamma ==
  <Theta> : Inport
  <Alpha> : Inport  Port=2
  Add : Sum  Inputs=+-
  Atan2 : Trigonometry  Operator=atan2
  Cos : Trigonometry  Operator=cos
  Cos1 : Trigonometry
  Out1 : Outport
  wires:
  Atan2/1 -> Out1/1
  <Alpha>/1 -> Add/2
  Add/1 -> Cos1/1, Cos/1
  <Theta>/1 -> Add/1
  Cos1/1 -> Atan2/1
  Cos/1 -> Atan2/2

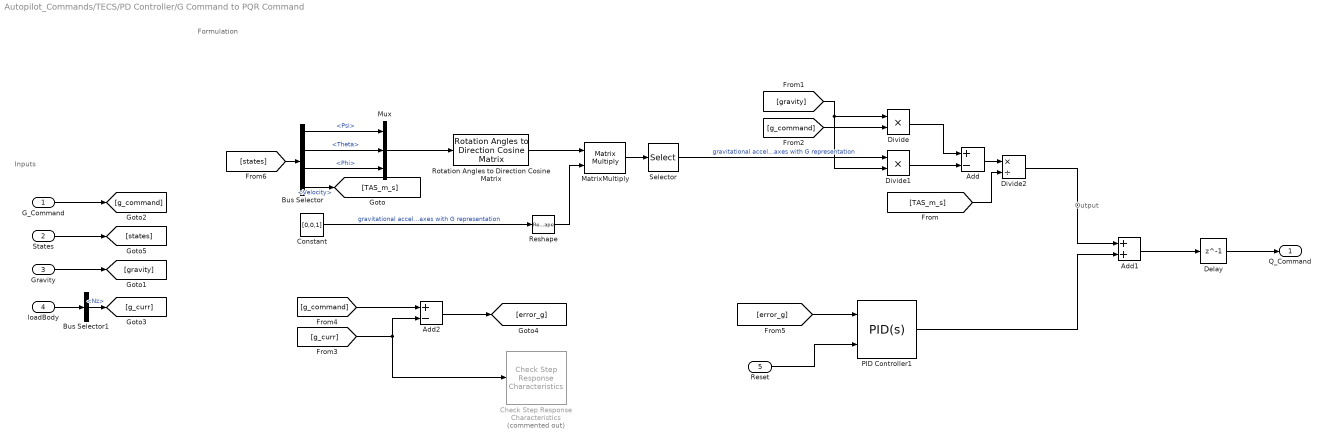
== system Autopilot_Commands/TECS/PD Controller/G Command to PQR Command ==
  note: Formulation
  note: Output
  note: Inputs
  G_Command : Inport
  States : Inport  Port=2
  Gravity : Inport  Port=3
  loadBody : Inport  Port=4
  Reset : Inport  Port=5
  Add : Sum  Inputs=+-
  Add1 : Sum
  Add2 : Sum  Inputs=+-
  Bus Selector : BusSelector  OutputSignals=Psi,Theta,Phi,Velocity
  Bus Selector1 : BusSelector  OutputSignals=Nz
  Check Step Response Characteristics : checkpacklib/Check Step Response  Characteristics  Commented=on  InstantiateOnLoad=on  enabled=off  stopWhenAssertionFail=off  export=off  ViewDlgPos=[]  OpenViewOnLoad=off  LaunchViewOnOpen=off  TimeUnits=seconds  EnableStepResponseBound=on  InitialValue=1  FinalValue=5  StepTime=0  RiseTime=0.5  PercentRise=90  SettlingTime=1.2  PercentSettling=1  PercentOvershoot=5  PercentUndershoot=1
      settings: LibrarySourceBlock=|
      | sdolib/Model Verification/Check Step Response
      | Characteristics
  Constant : Constant  Value=[0,0,1]
  Delay : Delay  DelayLength=1
  Divide : Product  Inputs=**
  Divide1 : Product  Inputs=**
  Divide2 : Product  Inputs=*/
  MatrixMultiply : Product  Multiplication=Matrix(*)
  Mux : Mux  Inputs=3
  PID Controller1 : slpidlib/PID Controller  Controller=PID  Form=Parallel  TimeDomain=Continuous-time  UseExternalTs=off  SampleTime=-1  IntegratorMethod=Forward Euler  FilterMethod=Forward Euler  ControllerParametersSource=internal  P=Kp  I=Ki  UseKiTs=off  D=Kd  N=100  UseFilter=on  TunerSelectOption=Transfer Function Based (PID Tuner App)  InitialConditionSource=internal  InitialConditionForIntegrator=0  InitialConditionForFilter=0  DifferentiatorICPrevScaledInput=0  ExternalReset=either  TrackingMode=off  Kt=1  LimitOutput=off  SatLimitsSource=external  UpperSaturationLimit=inf  LowerSaturationLimit=-inf  LinearizeAsGain=on  AntiWindupMode=clamping  Kb=1  LimitIntegrator=off  UpperIntegratorSaturationLimit=inf  LowerIntegratorSaturationLimit=-inf  POutMin=[]  POutMax=[]  IOutMin=[]  IOutMax=[]  DOutMin=[]  DOutMax=[]  NOutMin=[]  NOutMax=[]  SumOutMin=[]  SumOutMax=[]  SaturationOutMin=[]  SaturationOutMax=[]  PParamMin=[]  PParamMax=[]  IParamMin=[]  IParamMax=[]  DParamMin=[]  DParamMax=[]  NParamMin=[]  NParamMax=[]  KbParamMin=[]  KbParamMax=[]  KtParamMin=[]  KtParamMax=[]  KbOutMin=[]  KbOutMax=[]  KtOutMin=[]  KtOutMax=[]  IntegratorOutMin=[]  IntegratorOutMax=[]  FilterOutMin=[]  FilterOutMax=[]  SumI1OutMin=[]  SumI1OutMax=[]  SumI2OutMin=[]  SumI2OutMax=[]  SumI3OutMin=[]  SumI3OutMax=[]  SumI4OutMin=[]  SumI4OutMax=[]  SumDOutMin=[]  SumDOutMax=[]  DifferentiatorOutMin=[]  DifferentiatorOutMax=[]  FilterDiffOutCoefMin=[]  FilterDiffOutCoefMax=[]  ReciprocalOutMin=[]  ReciprocalOutMax=[]  SumDenOutMin=[]  SumDenOutMax=[]  SumNumOutMin=[]  SumNumOutMax=[]  DivideOutMin=[]  DivideOutMax=[]  UdiffTsProdOutMin=[]  UdiffTsProdOutMax=[]  NTsProdOutMin=[]  NTsProdOutMax=[]  UintegralTsProdOutMin=[]  UintegralTsProdOutMax=[]  UngainTsProdOutMin=[]  UngainTsProdOutMax=[]  ClampingZeroOutDataTypeStr=Inherit: Inherit via back propagation  ClampingZeroOutMin=[]  ClampingZeroOutMax=[]  FilterDenConstantOutDataTypeStr=Inherit: Inherit via back propagation  FilterDenConstantOutMin=[]  FilterDenConstantOutMax=[]  PCopyOutDataTypeStr=Inherit: Inherit via back propagation  PCopyOutMin=[]  PCopyOutMax=[]  NCopyOutDataTypeStr=Inherit: Inherit via back propagation  NCopyOutMin=[]  NCopyOutMax=[]  IntegratorContinuousStateAttributes=''  IntegratorStateMustResolveToSignalObject=off  IntegratorRTWStateStorageClass=Auto  FilterContinuousStateAttributes=''  FilterStateMustResolveToSignalObject=off  FilterRTWStateStorageClass=Auto  ParallelPVariant=InternalParameters  IdealPVariant=Disabled  IVariant=InternalParameters  DVariant=InternalParameters  IntegratorVariant=Continuous  SatVariant=Disabled  AWVariant=Passthrough  PCopyVariant=Disabled  TRVariant=Disabled  FdbkBlocksVariant=Forward  IdealPFdbkVariant=Disabled  SatFdbkVariant=Disabled  DerivativeFilterVariant=ContFilter  NVariant=InternalParameters  NCopyVariant=Disabled  FilterICVariant=InternalICsFilter  IntegratorICVariant=InternalICs  ExternalResetVariant=ExternalReset  TRSumVariant=Passthrough  SumFdbkVariant=Disabled  SumVariant=Sum_PID  TsampFilterVariant=InternalTs  TsampNgainVariant=Passthrough  TsampIntegralVariant=Disabled_SignalSpec  ExternalSaturationOutDataTypeStr=Inherit: Same as second input
  Reshape : Reshape  OutputDimensionality=Column vector (2-D)
  Rotation Angles to Direction Cosine Matrix : sharedtransform/Rotation Angles to Direction Cosine Matrix  rotationOrder=ZYX  aMode=aMode
  Selector : Selector  InputPortWidth=3  IndexOptions=Index vector (dialog)  Indices=3  OutputSizes=1
  Q_Command : Outport
  wires:
  [states] -> Bus Selector/1
  Delay/1 -> Q_Command/1
  Add2/1 -> [error_g]
  [g_curr] -> Add2/2, Check Step Response Characteristics/1
  [g_command] -> Add2/1
  Bus Selector1/1 -> [g_curr]  "<Nz>"
  loadBody/1 -> Bus Selector1/1
  Add1/1 -> Delay/1
  PID Controller1/1 -> Add1/2
  Reset/1 -> PID Controller1/2
  [error_g] -> PID Controller1/1
  G_Command/1 -> [g_command]
  Gravity/1 -> [gravity]
  Divide2/1 -> Add1/1
  Divide1/1 -> Add/2
  Divide/1 -> Add/1
  Selector/1 -> Divide1/1  "gravitational acceleration on Body Z axes with G representation"
  Add/1 -> Divide2/1
  [gravity] -> Divide1/2, Divide/1
  Reshape/1 -> MatrixMultiply/2
  [TAS_m_s] -> Divide2/2
  Bus Selector/4 -> [TAS_m_s]  "<Velocity>"
  [g_command] -> Divide/2
  MatrixMultiply/1 -> Selector/1
  Constant/1 -> Reshape/1  "gravitational acceleration on NED axes with G representation"
  Bus Selector/3 -> Mux/3  "<Phi>"
  Bus Selector/1 -> Mux/1  "<Psi>"
  Bus Selector/2 -> Mux/2  "<Theta>"
  Rotation Angles to Direction Cosine Matrix/1 -> MatrixMultiply/1
  Mux/1 -> Rotation Angles to Direction Cosine Matrix/1
  States/1 -> [states]
